simulink model "three_phase_inverter"  (R2013a)
settings: Solver=ode45  StartTime=0.0  StopTime=1  RelTol=1e-3
undefined symbols (not defined in the file): m
libraries: powerlib x13, powerlib_meascontrol x2, simulink x1
settings Model: Creator=TELE  LastModifiedBy=TELE

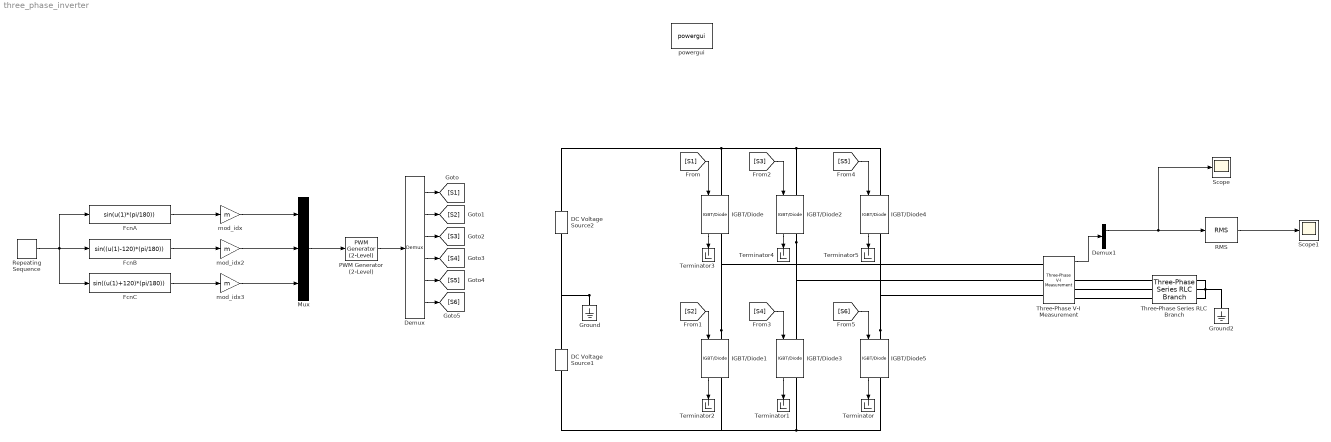
== system three_phase_inverter ==
  DC Voltage Source1 : powerlib/Electrical Sources/DC Voltage Source  Amplitude=200  Measurements=None
  DC Voltage Source2 : powerlib/Electrical Sources/DC Voltage Source  Amplitude=200  Measurements=None
  Demux : Demux  Outputs=6
  Demux1 : Demux  Outputs=3
  FcnA : Fcn  Expr=sin(u(1)*(pi/180))
  FcnB : Fcn  Expr=sin((u(1)-120)*(pi/180))
  FcnC : Fcn  Expr=sin((u(1)+120)*(pi/180))
  Ground : powerlib/Elements/Ground  LConnTagsString=a
  Ground2 : powerlib/Elements/Ground  LConnTagsString=a
  IGBT/Diode{,1..5} (6 alike) : powerlib/Power Electronics/IGBT//Diode  Ron=1e-3  Rs=1e5  Cs=inf  Measurements=on
  Mux : Mux  Inputs=3
  PWM Generator (2-Level) : powerlib_meascontrol/Pulse & Signal Generators/PWM Generator (2-Level)  ModulatorType=Three-phase bridge (6 pulses)  ModulatorMode=Unsynchronized  nF=27  Fc=27*50  ModulatingSignals=off  m=1  Freq=50  Phase=0  Ts=0
  RMS : powerlib_meascontrol/Measurements/RMS  TrueRMS=on  Freq=60  RMSInit=120  Ts=0
  Repeating Sequence : simulink/Sources/Repeating Sequence  rep_seq_t=[0 1/50]  rep_seq_y=[0 360]
  Scope : Scope
      settings: YMin=-225  YMax=225
  Scope1 : Scope
  Terminator{,1..5} (6 alike) : Terminator
  Three-Phase Series RLC Branch : powerlib/Elements/Three-Phase Series RLC Branch  LConnTagsString=A|B|C  RConnTagsString=A|B|C  BranchType=RLC  Resistance=10  Inductance=100e-3  Capacitance=1e-6  Measurements=None
  Three-Phase V-I Measurement : powerlib/Measurements/Three-Phase V-I Measurement  VoltageMeasurement=phase-to-ground  SetLabelV=off  LabelV=Vabc  Vpu=off  VpuLL=off  CurrentMeasurement=yes  SetLabelI=off  LabelI=Iabc  Ipu=off  Pbase=100e6  Vbase=500e3  OutputType=Complex  PhasorSimulation=off  PSBequivalent=0
  "mod_idx " : Gain  Gain=m
  mod_idx2 : Gain  Gain=m
  mod_idx3 : Gain  Gain=m
  powergui : powerlib/powergui  Priority=1  SimulationMode=Discrete  SolverType=Tustin  SampleTime=50e-6  frequency=60  SPID=off  DisableSnubberDevices=off  DisableRonSwitches=off  DisableVfSwitches=off  SwTol=0  Interpol=off  DisplayEquations=off  frequencyindice=0  Pbase=100e6  ErrMax=1e-4  Iterations=50  UnitsV=kV  UnitsW=MW  FunctionMessages=off  echomessages=off  HookPort=off  EnableUseOfTLC=off  x0status=blocks  RestoreLinks=warning  ResistiveCurrentMeasurement=off  Frange=[0:2:500]  Ylog=off  Xlog=on  ShowGrid=off  save=off  variable=ZData  ZoomFFT=off  StartTime=0.0  cycles=1  DisplayStyle=1  fundamental=60  FreqAxis=off  MaxFrequency=1000  frequencyindicesteady=1  RmsSteady=1  display=off  Ts=0  methode=off
  wires:
  Demux/1 -> [S1]
  Demux/2 -> [S2]
  Demux/3 -> [S3]
  Demux/4 -> [S4]
  Demux/5 -> [S5]
  Demux/6 -> [S6]
  PWM Generator (2-Level)/1 -> Demux/1
  FcnA/1 -> "mod_idx "/1
  FcnB/1 -> mod_idx2/1
  FcnC/1 -> mod_idx3/1
  Three-Phase V-I Measurement/1 -> Demux1/1
  Demux1/1 -> RMS/1, Scope/1
  RMS/1 -> Scope1/1
  Mux/1 -> PWM Generator (2-Level)/1
  Repeating Sequence/1 -> FcnA/1, FcnC/1, FcnB/1
  "mod_idx "/1 -> Mux/1
  mod_idx2/1 -> Mux/2
  mod_idx3/1 -> Mux/3
  [S6] -> IGBT/Diode5/1
  IGBT/Diode5/1 -> Terminator/1
  IGBT/Diode/1 -> Terminator3/1
  [S1] -> IGBT/Diode/1
  IGBT/Diode2/1 -> Terminator4/1
  IGBT/Diode3/1 -> Terminator1/1
  [S4] -> IGBT/Diode3/1
  [S2] -> IGBT/Diode1/1
  [S5] -> IGBT/Diode4/1
  IGBT/Diode4/1 -> Terminator5/1
  [S3] -> IGBT/Diode2/1
  IGBT/Diode1/1 -> Terminator2/1
  connections:
  Three-Phase Series RLC Branch/RConn1 -- Ground2/LConn1 -- Three-Phase Series RLC Branch/RConn2 -- Three-Phase Series RLC Branch/RConn3
  Three-Phase V-I Measurement/RConn2 -- Three-Phase Series RLC Branch/LConn2
  Three-Phase Series RLC Branch/LConn1 -- Three-Phase V-I Measurement/RConn1
  Three-Phase Series RLC Branch/LConn3 -- Three-Phase V-I Measurement/RConn3
  IGBT/Diode1/LConn1 -- Three-Phase V-I Measurement/LConn1 -- IGBT/Diode/RConn1
  IGBT/Diode5/LConn1 -- Three-Phase V-I Measurement/LConn3 -- IGBT/Diode4/RConn1
  IGBT/Diode/LConn1 -- DC Voltage Source2/RConn1 -- IGBT/Diode4/LConn1 -- IGBT/Diode2/LConn1
  Ground/LConn1 -- DC Voltage Source2/LConn1 -- DC Voltage Source1/RConn1
  IGBT/Diode3/RConn1 -- IGBT/Diode5/RConn1 -- IGBT/Diode1/RConn1 -- DC Voltage Source1/LConn1
  IGBT/Diode2/RConn1 -- Three-Phase V-I Measurement/LConn2 -- IGBT/Diode3/LConn1
